simulink library "mylib2"  (R2021a)
settings: Solver=VariableStepDiscrete  StartTime=0.0  StopTime=10.0  RelTol=1e-3  EnableMultiTasking=on
libraries: dsparch4 x1
settings Model: Creator=bbhattac  LastModifiedBy=LiPhoebe
settings SolverCC: AlgebraicLoopSolver=TrustRegion
settings DataIOCC: LimitDataPoints=on  SaveFormat=Array  ReturnWorkspaceOutputs=off
settings OptimizationCC: ExpressionDepthLimit=2147483647  LifeSpan=inf
settings DebuggingCC: UnderspecifiedInitializationDetection=Classic  MergeDetectMultiDrivingBlocksExec=none  SolverPrmCheckMsg=warning  ParameterPrecisionLossMsg=none  FcnCallInpInsideContextMsg=warning  StateNameClashWarn=warning  SFUnexpectedBacktrackingDiag=warning  SFNoUnconditionalDefaultTransitionDiag=warning  SFExecutionAtInitializationDiag=none  SFMachineParentedDataDiag=warning  ArithmeticOperatorsInVariantConditions=warning
settings HardwareCC: ProdBitPerPointer=32  ProdBitPerSizeT=32  ProdBitPerPtrDiffT=32  ProdLargestAtomicFloat=None  ProdIntDivRoundTo=Undefined  ProdEndianess=Unspecified  ProdWordSize=32  ProdHWDeviceType=32-bit Generic
settings ModelReferenceCC: PropagateSignalLabelsOutOfModel=off
settings SFSimCC: SimUseLocalCustomCode=off  CustomCodeUndefinedFunction=UseInterfaceOnly
settings RTWCC: RTWUseLocalCustomCode=off
settings CodeAppCC: StateflowObjectComments=on
settings GRTTargetCC: TargetLangStandard=C89/C90 (ANSI)  CombineOutputUpdateFcns=off  GRTInterface=on
settings ConfigComp: CovMetricSettings=dw  CovSaveCumulativeToWorkspaceVar=on  CovSaveSingleToWorkspaceVar=on  CovExternalEMLEnable=off

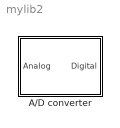
== system mylib2 ==
  A/D converter : Subsystem  mask(A/D converter){minDelay=1.0e-09, maxDelay=15.0e-09, nonlingain=0.2, nbits=8}
      mask prompts: minDelay "Minimum aperture delay"; maxDelay "Maximum aperture delay"; nonlingain "Nonlinear gain"; nbits "No. of quantization bits"
      mask help: Simulates typical ADC impairments. Mask parameters control the degree of impairment simulated by the block.
      mask init:
      | stepsize = 2^(-nbits);
      mask Help:
      | Minimum aperture delay and Maximum aperture delay: These control the aperture jitter for the ADC.
      | 
      | Nonlinear gain: This parameter controls the amount of nonlinear distortion in the ADC transfer function.
      | 
      | No. of quantization bits: Specifies the number of quantization bits for the ADC.
      mask Display:
      | plot([0,1,1,2,2,3,3,4,4],[0,0,1,1,2,2,3,3,4]);
      | plot([0,4],[2,2]);
      | plot([2,2],[0,4]);
      | % Note that you don't need to specify 'hold on'
      | % to keep plotting on the same axis for the icon.
      | text(0.3,3,'ADC');

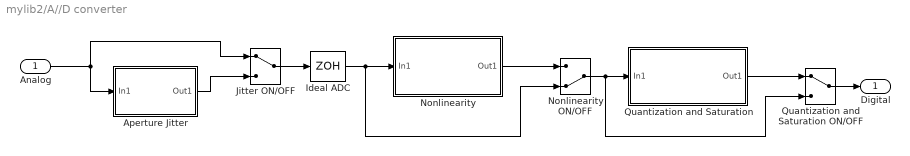
== system mylib2/A//D converter ==
  Analog : Inport
  Aperture Jitter : Subsystem
  Ideal ADC : ZeroOrderHold  SampleTime=1/100e6
  Jitter ON/OFF : ManualSwitch
  Nonlinearity : Subsystem
  Nonlinearity ON/OFF : ManualSwitch  CurrentSetting=0
  Quantization and Saturation ON/OFF : ManualSwitch
  Quantization and Saturation : Subsystem
  Digital : Outport  VectorParamsAs1DForOutWhenUnconnected=off
  wires:
  Analog/1 -> Jitter ON/OFF/1, Aperture Jitter/1(In1)
  Jitter ON/OFF/1 -> Ideal ADC/1
  Ideal ADC/1 -> Nonlinearity ON/OFF/2, Nonlinearity/1(In1)
  Quantization and Saturation/1(Out1) -> Quantization and Saturation ON/OFF/1
  Nonlinearity ON/OFF/1 -> Quantization and Saturation ON/OFF/2, Quantization and Saturation/1(In1)
  Nonlinearity/1(Out1) -> Nonlinearity ON/OFF/1
  Quantization and Saturation ON/OFF/1 -> Digital/1
  Aperture Jitter/1(Out1) -> Jitter ON/OFF/2

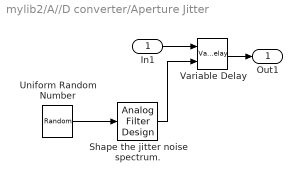
== system mylib2/A//D converter/Aperture Jitter ==
  In1 : Inport
  "Shape the jitter noise spectrum. " : dsparch4/Analog Filter Design  method=Butterworth  filttype=Lowpass  N=3  Wlo=2*pi*20e6  Whi=80  Rp=2  Rs=40
  Uniform Random Number : UniformRandomNumber  Minimum=minDelay  Maximum=maxDelay  Seed=1234  SampleTime=0
  Variable Delay : VariableTransportDelay  MaximumDelay=maxDelay  ZeroDelay=on  TransDelayFeedthrough=on
  Out1 : Outport  VectorParamsAs1DForOutWhenUnconnected=off
  wires:
  Uniform Random Number/1 -> "Shape the jitter noise spectrum. "/1
  "Shape the jitter noise spectrum. "/1 -> Variable Delay/2
  In1/1 -> Variable Delay/1
  Variable Delay/1 -> Out1/1

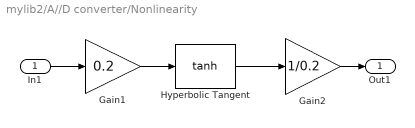
== system mylib2/A//D converter/Nonlinearity ==
  In1 : Inport
  Gain1 : Gain  Gain=0.2  SaturateOnIntegerOverflow=on  OutDataTypeStr=Inherit: Same as input  ParamDataTypeStr=Inherit: Same as input
  Gain2 : Gain  Gain=1/0.2  SaturateOnIntegerOverflow=on  OutDataTypeStr=Inherit: Same as input  ParamDataTypeStr=Inherit: Same as input
  Hyperbolic Tangent : Trigonometry  Operator=tanh
  Out1 : Outport  VectorParamsAs1DForOutWhenUnconnected=off
  wires:
  Hyperbolic Tangent/1 -> Gain2/1
  Gain1/1 -> Hyperbolic Tangent/1
  In1/1 -> Gain1/1
  Gain2/1 -> Out1/1

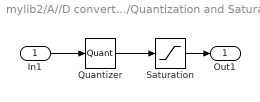
== system mylib2/A//D converter/Quantization and Saturation ==
  In1 : Inport
  Quantizer : Quantizer  QuantizationInterval=stepsize
  Saturation : Saturate  UpperLimit=1  LowerLimit=-1
  Out1 : Outport  VectorParamsAs1DForOutWhenUnconnected=off
  wires:
  Quantizer/1 -> Saturation/1
  In1/1 -> Quantizer/1
  Saturation/1 -> Out1/1
